simulink model "Laba_3"  (Simulink 9.2)
settings: Solver=ode45  StartTime=0.0  StopTime=10  RelTol=1e-3  EnableMultiTasking=on
settings Model: Creator=Vano  LastModifiedBy=murad
settings OptimizationCC: ExpressionDepthLimit=2147483647
settings DebuggingCC: SolverPrmCheckMsg=warning

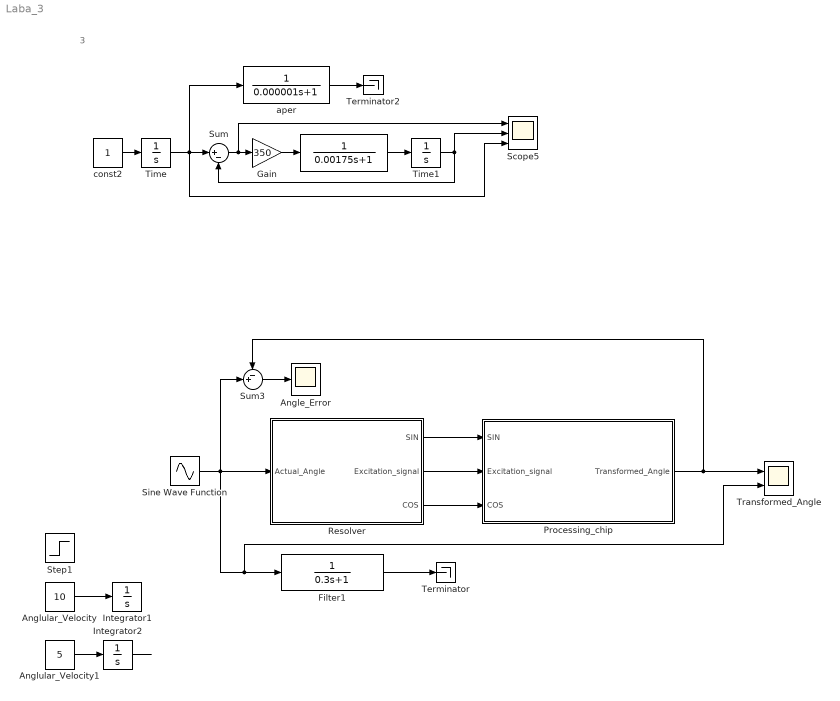
== system Laba_3 ==
  note: 3
  "  " : TransferFcn  Denominator=[0.00175 1]
  "Angle_Error " : Scope
  Anglular_Velocity : Constant  Value=10
  Anglular_Velocity1 : Constant  Value=5
  Filter1 : TransferFcn  Denominator=[0.3 1]
  Gain : Gain  Gain=350
  Integrator1 : Integrator
  Integrator2 : Integrator
  Processing_chip : Subsystem
  Resolver : Subsystem
  Scope5 : Scope  NumInputPorts=3
  Sine Wave Function : Sin  SampleTime=0
  Step1 : Step  Time=0.05  After=1.5  SampleTime=0
  Sum : Sum  Inputs=|+-
  Sum3 : Sum  Inputs=-+|
  Terminator : Terminator
  "Terminator2 " : Terminator
  "Time " : Integrator
  Time1 : Integrator
  "Transformed_Angle " : Scope  NumInputPorts=2
  aper : TransferFcn  Denominator=[0.000001 1]
  const2 : Constant
  wires:
  "Time "/1 -> aper/1, Scope5/3, Sum/1
  const2/1 -> "Time "/1
  aper/1 -> "Terminator2 "/1
  "  "/1 -> Time1/1
  Gain/1 -> "  "/1
  Sum/1 -> Scope5/1, Gain/1
  Time1/1 -> Sum/2, Scope5/2
  Sum3/1 -> "Angle_Error "/1
  Processing_chip/1(Transformed_Angle) -> "Transformed_Angle "/1, Sum3/1
  Filter1/1 -> Terminator/1
  Resolver/1(SIN) -> Processing_chip/1(SIN)
  Resolver/2(Excitation_signal) -> Processing_chip/2(Excitation_signal)
  Resolver/3(COS) -> Processing_chip/3(COS)
  Anglular_Velocity/1 -> Integrator1/1
  Sine Wave Function/1 -> Filter1/1, "Transformed_Angle "/2, Sum3/2, Resolver/1(Actual_Angle)
  Integrator2/1 -> ?
  Anglular_Velocity1/1 -> Integrator2/1

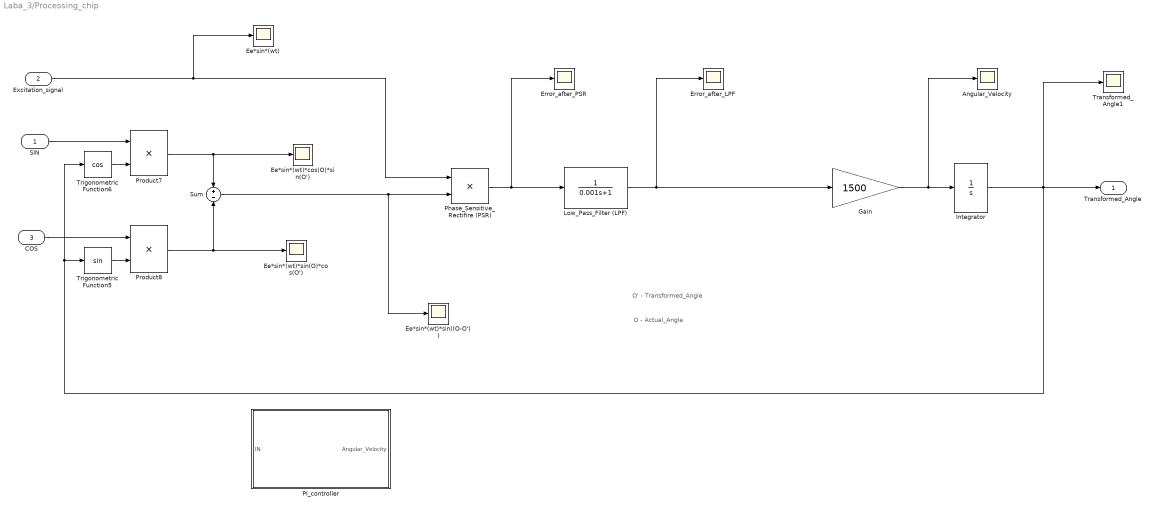
== system Laba_3/Processing_chip ==
  note: O' - Transformed_Angle
  note: O - Actual_Angle
  SIN : Inport
  Excitation_signal : Inport  Port=2
  COS : Inport  Port=3
  Angular_Velocity : Scope
  Ee*sin*(wt) : Scope
  Ee*sin*(wt)*cos(O)*sin(O') : Scope
  Ee*sin*(wt)*sin((O-O')) : Scope
  Ee*sin*(wt)*sin(O)*cos(O') : Scope
  Error_after_LPF : Scope
  Error_after_PSR : Scope
  Gain : Gain  Gain=1500
  Integrator : Integrator
  Low_Pass_Filter (LPF) : TransferFcn  Denominator=[0.001 1]
  PI_controller : Subsystem
  Phase_Sensitive_Rectifire (PSR) : Product  RndMeth=Zero
  Product7 : Product  RndMeth=Zero
  Product8 : Product  RndMeth=Zero
  Sum : Sum  Inputs=+-
  Transformed_Angle1 : Scope
  Trigonometric Function5 : Trigonometry
  Trigonometric Function6 : Trigonometry  Operator=cos
  Transformed_Angle : Outport
  wires:
  Trigonometric Function6/1 -> Product7/2
  Trigonometric Function5/1 -> Product8/2
  Product7/1 -> Sum/1, Ee*sin*(wt)*cos(O)*sin(O')/1
  Product8/1 -> Sum/2, Ee*sin*(wt)*sin(O)*cos(O')/1
  SIN/1 -> Product7/1
  COS/1 -> Product8/1
  Excitation_signal/1 -> Phase_Sensitive_Rectifire (PSR)/1, Ee*sin*(wt)/1
  Phase_Sensitive_Rectifire (PSR)/1 -> Low_Pass_Filter (LPF)/1, Error_after_PSR/1
  Sum/1 -> Phase_Sensitive_Rectifire (PSR)/2, Ee*sin*(wt)*sin((O-O'))/1
  Gain/1 -> Integrator/1, Angular_Velocity/1
  Integrator/1 -> Transformed_Angle1/1, Trigonometric Function5/1, Trigonometric Function6/1, Transformed_Angle/1
  Low_Pass_Filter (LPF)/1 -> Gain/1, Error_after_LPF/1

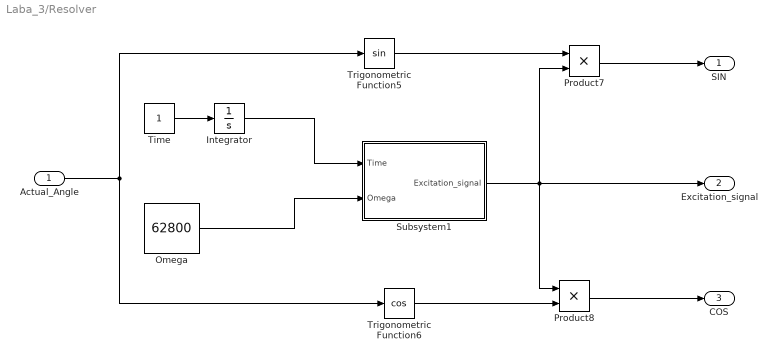
== system Laba_3/Resolver ==
  Actual_Angle : Inport
  Integrator : Integrator
  Omega : Constant  Value=62800
  Product7 : Product  RndMeth=Zero
  Product8 : Product  RndMeth=Zero
  Subsystem1 : Subsystem
  Time : Constant
  Trigonometric Function5 : Trigonometry
  Trigonometric Function6 : Trigonometry  Operator=cos
  SIN : Outport
  Excitation_signal : Outport  Port=2
  COS : Outport  Port=3
  wires:
  Time/1 -> Integrator/1
  Integrator/1 -> Subsystem1/1(Time)
  Omega/1 -> Subsystem1/2(Omega)
  Actual_Angle/1 -> Trigonometric Function6/1, Trigonometric Function5/1
  Trigonometric Function6/1 -> Product8/2
  Trigonometric Function5/1 -> Product7/1
  Subsystem1/1(Excitation_signal) -> Product7/2, Product8/1, Excitation_signal/1
  Product7/1 -> SIN/1
  Product8/1 -> COS/1

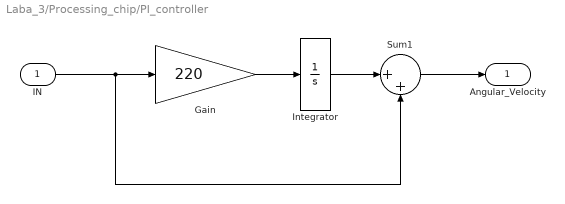
== system Laba_3/Processing_chip/PI_controller ==
  IN : Inport
  Gain : Gain  Gain=220
  Integrator : Integrator
  Sum1 : Sum  Inputs=|++
  Angular_Velocity : Outport
  wires:
  Sum1/1 -> Angular_Velocity/1
  IN/1 -> Sum1/2, Gain/1
  Integrator/1 -> Sum1/1
  Gain/1 -> Integrator/1

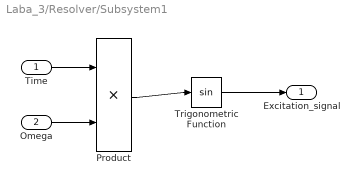
== system Laba_3/Resolver/Subsystem1 ==
  Time : Inport
  Omega : Inport  Port=2
  Product : Product  RndMeth=Zero
  Trigonometric Function : Trigonometry
  Excitation_signal : Outport
  wires:
  Omega/1 -> Product/2
  Trigonometric Function/1 -> Excitation_signal/1
  Time/1 -> Product/1
  Product/1 -> Trigonometric Function/1
